simulink model "WIP_2g"  (R2025b)
settings: Solver=ode15s  StartTime=0.0  StopTime=100  MaxStep=1e-2  RelTol=1e-6
InitFcn:
  | run("init.m");
values from neighbouring files (symbols this model uses):
  Fast_Ts = 1e-4    (= 0.0001)    [init.m]
  K1 = robot_params.m1  * robot_params.lc1 + (robot_params.m2 + robot_params.meq)*robot_params.l1    [init.m]
  K2 = robot_params.m2  * robot_params.lc2 + robot_params.meq*robot_params.l2    [init.m]
  q1_init = 0.01; -pi/42;0.01    [init.m]
  q2_init = asin(-K1/K2*sin(q1_init))    [init.m]
undefined symbols (not defined in the file or in its folder): robot_params
settings Model: Creator=Acer  LastModifiedBy=Acer
settings SolverCC: InitialStep=1e-5  SolverResetMethod=Robust

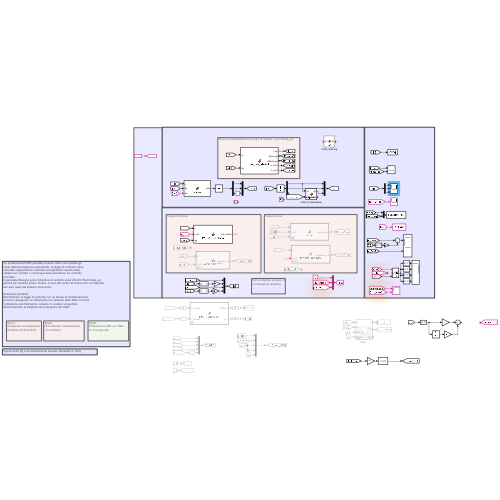
[thumbnail: Simulink's stored preview of the top-level diagram]
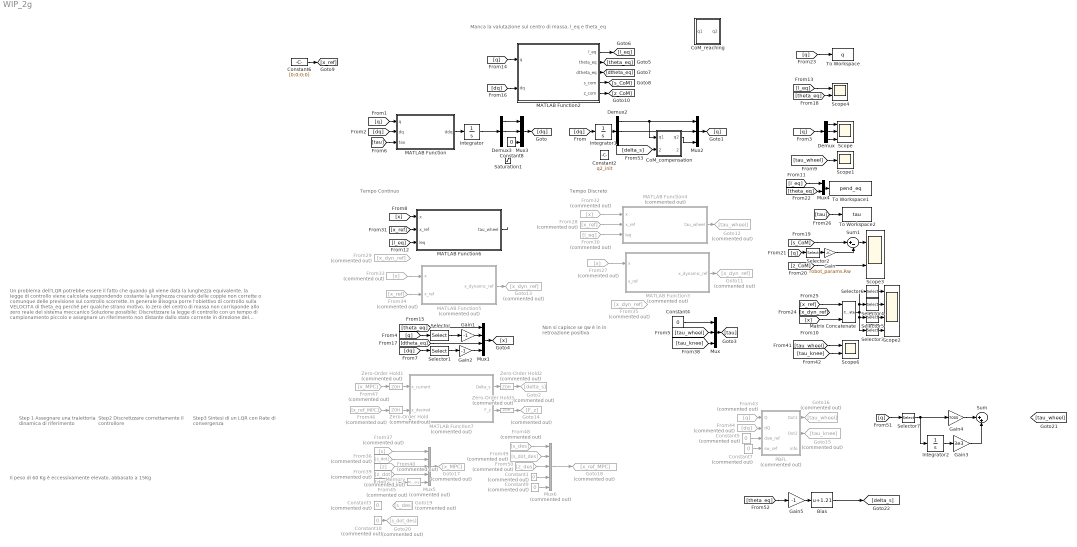
== system WIP_2g ==
  note: Non si capisce se qw è in
      | in retroazione positiva
  note: Il peso di 60 Kg è eccessivamente elevato, abbasato a 15Kg
  note: Tempo Continuo
  note: Step 1
      | Assegnare una traiettoria
      | dinamica di riferimento
  note: Un problema dell'LQR potrebbe essere il fatto che quando gli
      | viene data la lunghezza equivalente, la legge di controllo viene
      | calcolata suppondendo costante la lunghezza creando delle
      | coppie non corrette o comunque delle previsione sul controllo
      | scorrette.
      | In generale Bisogna porre l'obiettivo di controllo sulla VELOCITA di theta_eq
      | perché per qualche strano motivo, lo zero del centro di massa non corrisponde
      | allo zero reale del sistema meccanico
      |
      | Soluzione possibile:
      | Discretizzare la legge di controllo con un tempo di campionamento
      | piccolo e assegnare un riferimento non distante dallo stato corrente
      | in direzione del riferimento costante. In soldoni: progettare
      | dinamicamente la traiettoria da assegnare allo stato
  note: Manca la valutazione sul centro di massa, l_eq e theta_eq
  note: Step2
      | Discretizzare correttamente
      |  il controllore
  note: Tempo Discreto
  note: Step3
      | Sintesi di un LQR con Rate
      | di convergenza
  Bias : Bias  Bias=1.21  SaturateOnIntegerOverflow=off
  CoM_compensation : MATLAB Function  TreatAsAtomicUnit=on
  CoM_reaching : MATLAB Function  TreatAsAtomicUnit=on
  Constant{1,3,5,7,9..10} (6 alike) : Constant  Commented=on  Value=0
  Constant2 : Constant  Value=q2_init
  Constant4 : Constant  Value=0
  Constant6 : Constant  Value=[0;0;0;0]
  Constant8 : Constant  Value=0
  Demux : Demux  Outputs=3
  Demux2 : Demux  Outputs=3
  Demux3 : Demux  Outputs=3
  From27 : From  Commented=on  GotoTag=x
  From28 : From  Commented=on  GotoTag=x_ref
  From29 : From  Commented=on  GotoTag=x_dyn_ref
  From30 : From  Commented=on  GotoTag=l_eq
  From32 : From  Commented=on  GotoTag=x
  From33 : From  Commented=on  GotoTag=x
  From34 : From  Commented=on  GotoTag=x_ref
  From35 : From  Commented=on  GotoTag=x_dyn_ref
  From36 : From  Commented=on  GotoTag=s_dot
  From37 : From  Commented=on  GotoTag=s
  From39 : From  Commented=on  GotoTag=z_dot
  From40 : From  Commented=on  GotoTag=z
  From43 : From  Commented=on  GotoTag=q
  From44 : From  Commented=on  GotoTag=dq
  From45 : From  Commented=on  GotoTag=delta_s
  From46 : From  Commented=on  GotoTag=x_ref_MPC
  From47 : From  Commented=on  GotoTag=x_MPC
  From48 : From  Commented=on  GotoTag=s_des
  From49 : From  Commented=on  GotoTag=s_dot_des
  From50 : From  Commented=on  GotoTag=z_des
  Gain : Gain  Gain=robot_params.Rw
  Gain1 : Gain  Gain=-1
  Gain2 : Gain  Gain=-1
  Gain3 : Gain  Gain=3e3
  Gain4 : Gain  Gain=7000
  Gain5 : Gain  Gain=-1
  Goto11 : Goto  Commented=on  GotoTag=x_dyn_ref
  Goto12 : Goto  Commented=on  GotoTag=tau_wheel
  Goto13 : Goto  Commented=on  GotoTag=x_dyn_ref
  Goto14 : Goto  Commented=on  GotoTag=F_z
  Goto15 : Goto  Commented=on  GotoTag=tau_knee
  Goto16 : Goto  Commented=on  GotoTag=tau_wheel
  Goto17 : Goto  Commented=on  GotoTag=x_MPC
  Goto18 : Goto  Commented=on  GotoTag=x_ref_MPC
  Goto19 : Goto  Commented=on  GotoTag=s_des
  Goto2 : Goto  Commented=on  GotoTag=delta_s
  Goto20 : Goto  Commented=on  GotoTag=s_dot_des
  Integrator : Integrator  InitialCondition=[0;0;0]  ContinuousStateAttributes="\"dq\""
  Integrator1 : Integrator  InitialCondition=[q1_init;0;q2_init]  ContinuousStateAttributes="\"q\""
  Integrator2 : Integrator
  MATLAB Function : MATLAB Function  TreatAsAtomicUnit=on
  MATLAB Function2 : MATLAB Function  TreatAsAtomicUnit=on
  MATLAB Function3 : MATLAB Function  Commented=on  TreatAsAtomicUnit=on  mask{nTs=10, max_amplification=100, min_amplification=1e-3}
  MATLAB Function4 : MATLAB Function  Commented=on  TreatAsAtomicUnit=on
  MATLAB Function5 : MATLAB Function  Commented=on  TreatAsAtomicUnit=on  mask{nTs=1.5, max_amplification=100, min_amplification=1e-3}
  MATLAB Function6 : MATLAB Function  TreatAsAtomicUnit=on  mask{t_settling=10, Q=[1e-10, 1e-10,1e6,1e-3]}
  MATLAB Function7 : MATLAB Function  Commented=on  TreatAsAtomicUnit=on
  Matrix Concatenate : Concatenate  NumInputs=3  Mode=Multidimensional array  ConcatenateDimension=2
  Memory : Memory  Commented=on
  Mux : Mux  Inputs=3
  Mux1 : Mux
  Mux2 : Mux  Inputs=3
  Mux3 : Mux  Inputs=3
  Mux4 : Mux  Inputs=2
  Mux5 : Mux  Commented=on  Inputs=5
  Mux6 : Mux  Commented=on  Inputs=5
  PBFL : Subsystem  Commented=on
  Saturation1 : Saturate  UpperLimit=1  LowerLimit=-1
  Scope : Scope  NumInputPorts=3
      settings: ActiveDisplayString=3  Title=q2  ActiveDisplayYMinimum=1.570486578406654  ActiveDisplayYMaximum=1.5708307432824791
  Scope1 : Scope
      settings: ActiveDisplayYMinimum=-114.88856363268619  ActiveDisplayYMaximum=34.027418421979604
  Scope2 : Scope  NumInputPorts=4
      settings: ActiveDisplayString=4  Title=dqw  ActiveDisplayYMinimum=-52.982971865328068  ActiveDisplayYMaximum=78.205633765029773  DataLoggingVariableName=ScopeData2
  Scope3 : Scope  NumInputPorts=2
      settings: Title=s_CoM - s  ActiveDisplayYMinimum=-0.00016761515520245026  ActiveDisplayYMaximum=1.8924319875646953E-5  DataLoggingVariableName=ScopeData3
  Scope4 : Scope  NumInputPorts=2
      settings: Title=theta_eq  ActiveDisplayYMinimum=-5.3281452597715081E-16  ActiveDisplayYMaximum=4.7823411124945276E-16  DataLoggingVariableName=ScopeData4
  Scope6 : Scope  NumInputPorts=2
      settings: Title=tau_knee  ActiveDisplayYMinimum=-39.904031097666696  ActiveDisplayYMaximum=17.79706307326623  DataLoggingVariableName=ScopeData6
  Selector : Selector  InputPortWidth=3  IndexOptions=Index vector (dialog)  Indices=[2]  OutputSizes=1
  Selector1 : Selector  InputPortWidth=3  IndexOptions=Index vector (dialog)  Indices=[2]  OutputSizes=1
  Selector2 : Selector  InputPortWidth=3  IndexOptions=Index vector (dialog)  Indices=[2]  OutputSizes=1
  Selector3 : Selector  NumberOfDimensions=2  InputPortWidth=3  IndexOptions=Index vector (dialog),Index vector (dialog)  Indices=[4],[1 2 3]  OutputSizes=1,1
  Selector4 : Selector  NumberOfDimensions=2  InputPortWidth=3  IndexOptions=Index vector (dialog),Index vector (dialog)  Indices=[2],[1 2 3]  OutputSizes=1,1
  Selector5 : Selector  NumberOfDimensions=2  InputPortWidth=3  IndexOptions=Index vector (dialog),Index vector (dialog)  Indices=[3],[1 2 3]  OutputSizes=1,1
  Selector6 : Selector  NumberOfDimensions=2  InputPortWidth=3  IndexOptions=Index vector (dialog),Index vector (dialog)  Indices=[1],[1 2 3]  OutputSizes=1,1
  Selector7 : Selector  InputPortWidth=3  IndexOptions=Index vector (dialog)  Indices=1  OutputSizes=1
  Sum : Sum  Inputs=|++
  Sum1 : Sum  Inputs=|+-
  To Workspace : ToWorkspace  VariableName=q  SaveFormat=Timeseries  SampleTime=-1
  To Workspace1 : ToWorkspace  VariableName=pend_eq  SaveFormat=Timeseries  SampleTime=-1
  To Workspace2 : ToWorkspace  VariableName=tau  SaveFormat=Timeseries  SampleTime=-1
  Zero-Order Hold{,1..3} (4 alike) : ZeroOrderHold  Commented=on  SampleTime=1e-2
  wires:
  MATLAB Function/1(ddq) -> Integrator/1
  [dq] -> Integrator1/1
  [q] -> MATLAB Function/1(q)
  [dq] -> MATLAB Function/2(dq)
  Demux/1 -> Scope/1
  [q] -> Demux/1
  Demux/2 -> Scope/2
  [x_ref] -> MATLAB Function6/2(x_ref)
  [l_eq] -> MATLAB Function6/3(leq)
  [tau_wheel] -> Mux/2
  Constant4/1 -> Mux/1
  Mux/1 -> [tau]
  [q] -> Selector/1
  [dq] -> Selector1/1
  Mux1/1 -> [x]
  [x] -> MATLAB Function6/1(x)
  [tau_wheel] -> Scope1/1
  Selector6/1 -> Scope2/1
  Selector4/1 -> Scope2/2
  Selector5/1 -> Scope2/3
  Selector3/1 -> Scope2/4
  [l_eq] -> Scope4/1
  [tau_knee] -> Mux/3
  Demux/3 -> Scope/3
  Integrator1/1 -> Demux2/1
  Mux2/1 -> [q]
  Mux3/1 -> [dq]
  Integrator/1 -> Demux3/1
  [q] -> MATLAB Function2/1(q)
  MATLAB Function2/1(l_eq) -> [l_eq]
  MATLAB Function2/2(theta_eq) -> [theta_eq]
  [theta_eq] -> Mux1/1
  [dq] -> MATLAB Function2/2(dq)
  MATLAB Function2/3(dtheta_eq) -> [dtheta_eq]
  [dtheta_eq] -> Mux1/3
  [theta_eq] -> Scope4/2
  MATLAB Function2/4(s_com) -> [s_CoM]
  MATLAB Function2/5(z_com) -> [z_CoM]
  [s_CoM] -> Sum1/1
  [z_CoM] -> Scope3/2
  [q] -> Selector2/1
  Selector2/1 -> Gain/1
  Gain/1 -> Sum1/2
  Sum1/1 -> Scope3/1
  [theta_eq] -> Mux4/2
  [l_eq] -> Mux4/1
  Mux4/1 -> To Workspace1/1
  [q] -> To Workspace/1
  Constant6/1 -> [x_ref]
  From27/1 -> MATLAB Function3/1(x)
  MATLAB Function3/1(x_dynamic_ref) -> Goto11/1
  [x] -> Matrix Concatenate/3
  [x_ref] -> Matrix Concatenate/1
  Matrix Concatenate/1 -> Selector3/1, Selector5/1, Selector4/1, Selector6/1
  From32/1 -> MATLAB Function4/1(x)
  From30/1 -> MATLAB Function4/3(leq)
  From28/1 -> MATLAB Function4/2(x_ref)
  MATLAB Function5/1(x_dynamic_ref) -> Goto13/1
  From33/1 -> MATLAB Function5/1(x)
  From34/1 -> MATLAB Function5/2(x_ref)
  Selector/1 -> Gain1/1
  Gain1/1 -> Mux1/2
  Selector1/1 -> Gain2/1
  Gain2/1 -> Mux1/4
  ? -> MATLAB Function3/2(x_ref)
  [tau] -> To Workspace2/1
  [tau] -> MATLAB Function/3(tau)
  Demux3/2 -> Mux3/2
  Demux2/2 -> Mux2/2
  MATLAB Function4/1(tau_wheel) -> Goto12/1
  Demux2/1 -> CoM_compensation/1(q1), Mux2/1
  MATLAB Function6/1(tau_wheel) -> ?
  Demux3/1 -> Mux3/1
  [tau_wheel] -> Scope6/1
  [tau_knee] -> Scope6/2
  From43/1 -> PBFL/1(Q)
  From44/1 -> PBFL/2(dQ)
  Constant5/1 -> PBFL/3(dsw_ref)
  Constant7/1 -> PBFL/4(sw_ref)
  PBFL/1(Out1) -> Goto16/1
  PBFL/2(Out2) -> Goto15/1
  Constant8/1 -> Mux3/3
  CoM_compensation/1(q2) -> Mux2/3
  From47/1 -> Zero-Order Hold1/1
  From39/1 -> Mux5/4
  Zero-Order Hold3/1 -> Goto14/1
  Mux6/1 -> Goto18/1
  Memory/1 -> Mux5/5
  From46/1 -> Zero-Order Hold/1
  From48/1 -> Mux6/1
  MATLAB Function7/1(Delta_s) -> Zero-Order Hold2/1
  From50/1 -> Mux6/3
  Constant9/1 -> Mux6/5
  From36/1 -> Mux5/2
  From45/1 -> Memory/1
  From40/1 -> Mux5/3
  Zero-Order Hold1/1 -> MATLAB Function7/1(x_current)
  Zero-Order Hold/1 -> MATLAB Function7/2(x_desired)
  Constant1/1 -> Mux6/4
  From49/1 -> Mux6/2
  MATLAB Function7/2(F_z) -> Zero-Order Hold3/1
  From37/1 -> Mux5/1
  Zero-Order Hold2/1 -> Goto2/1
  Mux5/1 -> Goto17/1
  Constant10/1 -> Goto20/1
  [q] -> Selector7/1
  Gain4/1 -> Sum/1
  Gain3/1 -> Sum/2
  Integrator2/1 -> Gain3/1
  Selector7/1 -> Integrator2/1, Gain4/1
  [theta_eq] -> Gain5/1
  Gain5/1 -> Bias/1
  [delta_s] -> CoM_compensation/2(delta_s)
  Bias/1 -> [delta_s]

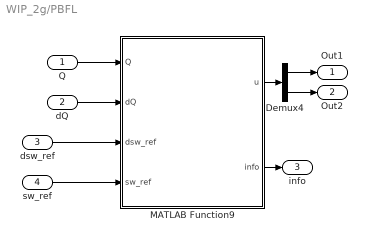
== system WIP_2g/PBFL ==
  Q : Inport
  dQ : Inport  Port=2
  dsw_ref : Inport  Port=3
  sw_ref : Inport  Port=4
  Demux4 : Demux  Outputs=2
  MATLAB Function9 : MATLAB Function  TreatAsAtomicUnit=on
  Out1 : Outport
  Out2 : Outport  Port=2
  info : Outport  Port=3
  wires:
  MATLAB Function9/1(u) -> Demux4/1
  Demux4/1 -> Out1/1
  dQ/1 -> MATLAB Function9/2(dQ)
  Q/1 -> MATLAB Function9/1(Q)
  Demux4/2 -> Out2/1
  MATLAB Function9/2(info) -> info/1
  sw_ref/1 -> MATLAB Function9/4(sw_ref)
  dsw_ref/1 -> MATLAB Function9/3(dsw_ref)

== matlab function WIP_2g/PBFL/MATLAB Function9 ==
  data: Q input; u output; dQ input; dsw_ref input; sw_ref input; info output; gains parameter
function [u, info] = pfl_biped_v3(Q, dQ, dsw_ref, sw_ref, gains)
%#codegen
% Tutti gli stati (Q, dQ) sono quelli reali del plant — nessun ingresso
% "virtuale" separato. theta_ref e' calcolato QUI dentro come funzione di
% qw, dqw, non e' un riferimento esterno fornito dall'utente.
%
% gains = [kp1; kd1; kp_pc; kd_pc; kv; kx; theta_max; pc_max; tau_max]

    Rw = 0.127;
    m1=1.2; m2=5.3; meq=15.0; l1=0.45; l2=0.45; lc1=l1/2; lc2=l2/2;
    K1 = m1*lc1 + (m2+meq)*l1;
    K2 = m2*lc2 + meq*l2;
    mtot = 3.5 + m1 + m2 + meq;

    kp1=gains(1); kd1=gains(2);
    kp_pc=gains(3); kd_pc=gains(4);
    kv=gains(5); kx=gains(6);
    theta_max=gains(7); pc_max=gains(8); tau_max=gains(9);

    q1=Q(1); qw=Q(2); q2=Q(3);
    dq1=dQ(1); dqw=dQ(2); dq2=dQ(3);
    c1=cos(q1); s1=sin(q1); c2=cos(q2); s2=sin(q2);

    [M,~,CdQ,G,B] = calc_dynamics(Q,dQ);
    h = CdQ + B*dQ + G;
    S = [-1,-1; 1,0; 0,1];

    % --- riferimento di postura DERIVATO dagli stati reali qw, dqw -------
    sw  = Rw*qw;
    dsw = Rw*dqw;
    theta_ref = -kv*(dsw - dsw_ref) - kx*(sw - sw_ref);
    theta_ref = sat(theta_ref, theta_max);

    % --- uscita 1: postura, ora rincorre theta_ref invece di una costante
    v1 = -kp1*(q1 - theta_ref) - kd1*dq1;

    % --- uscita 2: bilanciamento CoM, invariata -----------------------
    pc  = (K1*s1 + K2*s2)/mtot;
    dpc = (K1*c1*dq1 + K2*c2*dq2)/mtot;
    drift = -(K1*s1*dq1^2 + K2*s2*dq2^2)/mtot;
    pc_ref = sat(0, pc_max);   % qui puoi tenerlo a 0, il bilanciamento resta locale
    v2 = -kp_pc*(pc - pc_ref) - kd_pc*dpc;

    A = [1,0,0; K1*c1/mtot,0,K2*c2/mtot];
    D = A*(M\S);
    rhs = [v1; v2 - drift] + A*(M\h);

    u = D \ rhs;
    u = [sat(u(1),tau_max); sat(u(2),tau_max)];

    info = [theta_ref; pc; sw; dsw];
end

function y = sat(x,lim)
    y = min(max(x,-lim),lim);
end

== matlab function WIP_2g/MATLAB Function7 ==
  data: x_current input; Delta_s output; x_desired input; F_z output
function [Delta_s, F_z] = MPC_Custom_QP(x_current, x_desired)
    % quadprog non è supportato nativamente per la code generation C
    coder.extrinsic('quadprog');
    coder.extrinsic('optimoptions');

    %% 1. Parametri e Discretizzazione
    m_b = 73.0; 
    g = 9.81;    
    
    h = x_current(3); 
    if h < 0.1
        h = 0.6;
    end
    
    dt = 0.01; 
    N = 40;     
    
    A_c = zeros(5,5);
    A_c(1,2) = 1;
    A_c(3,4) = 1;
    A_c(2,5) = g / h; 
    
    B_c = zeros(5,2);
    B_c(4,2) = 1 / m_b;
    B_c(5,1) = 1;
    
    A_d = eye(5) + A_c * dt;
    B_d = B_c * dt;

    %% 2. Pesi della Funzione di Costo
    %x = [s, ṡ, z, ż, Δs]
    S = diag([1, 1, 500, 50, 1]);
    W = diag([1, 0.01]);

    %% 3. Condensazione (Srotolamento) 
    nx = 5; nu = 2;
    P_x = zeros(nx*N, nx);
    P_u = zeros(nx*N, nu*N);

    A_power = eye(nx);
    for i = 1:N
        A_power = A_power * A_d;
        P_x((i-1)*nx+1 : i*nx, :) = A_power;
        for j = 1:i
            P_u((i-1)*nx+1 : i*nx, (j-1)*nu+1 : j*nu) = (A_d^(i-j)) * B_d;
        end
    end

    S_bar = kron(eye(N), S);
    W_bar = kron(eye(N), W);

    H = 2 * (P_u' * S_bar * P_u + W_bar);
    H = (H + H') / 2; % Garantisce simmetria perfetta
    
    X_ref = repmat(x_desired, N, 1);
    f = 2 * P_u' * S_bar * (P_x * x_current - X_ref);

    %% 4. Vincoli Fisici
    F_min = -1500; % Permette di frenare!
    F_max = 1500;
    
    LB = zeros(nu*N, 1);
    UB = zeros(nu*N, 1);
    
    for i = 1:N
        LB((i-1)*nu+1) = -0.20;   % era -2.0

        UB((i-1)*nu+1) =  0.20;   % era  2.0
 
        
        LB((i-1)*nu+2) = F_min; 
        UB((i-1)*nu+2) = F_max;
    end

    %% 5. Risoluzione QP (CORRETTA)
    % Pre-allocazione per Simulink Coder
    U_opt_calc = zeros(nu*N, 1);
    fval = 0.0;
    exitflag = 0.0;
    
    % Algoritmo robusto di default
    options = optimoptions('quadprog', 'Display', 'off');
    
    % LA CORREZIONE: Aggiunto "fval" per non sballare "exitflag"!
    [U_opt_calc, fval, exitflag] = quadprog(H, f, [], [], [], [], LB, UB, [], options);

    if exitflag > 0
        U_opt = U_opt_calc;
    else
        % Se fallisce davvero, eroga 0 extra, ma il VMC ci terrà in piedi col peso base
        U_opt = zeros(nu*N, 1);
    end

    %% 6. Estrazione Input Ottimo
    Delta_s_dot_opt = U_opt(1);
    F_z = U_opt(2); % FINALMENTE SARA' DIVERSO DA ZERO!

    Delta_s = x_current(5) + Delta_s_dot_opt * dt;
end

== matlab function WIP_2g/MATLAB Function ==
  settings: updateMethod=CONTINUOUS
  data: q input double size=3; dq input double size=3; tau input size=3; ddq output double size=3; robot_params parameter
function ddq = Dynamics(q,dq,tau,robot_params)


q1 = q(1);
qw = q(2);
q2 = q(3);
dq1 = dq(1);
dqw = dq(2);
dq2 = dq(3);

m1 = robot_params.m1;
m2 = robot_params.m2;
meq = robot_params.meq;
lc2 = robot_params.lc1;
lc1 = robot_params.lc2;
l1 = robot_params.l1;
l2 = robot_params.l2;
mw = robot_params.mw;
Rw = robot_params.Rw;
Iw= robot_params.Iw;
g = robot_params.g;
bw =  robot_params.bw;
b1 =  robot_params.b1;
b2 = robot_params.b2;
I1 = robot_params.I1;  
I2 = robot_params.I2;



M = [ I1 + l1^2*m2 + lc1^2*m1 + l1^2*meq,        Rw*cos(q1)*(l1*m2 + lc1*m1 + l1*meq), l1*cos(q1 - q2)*(lc2*m2 + l2*meq);
      Rw*cos(q1)*(l1*m2 + lc1*m1 + l1*meq), Iw + Rw^2*m1 + Rw^2*m2 + Rw^2*meq + Rw^2*mw,      Rw*cos(q2)*(lc2*m2 + l2*meq);
       l1*cos(q1 - q2)*(lc2*m2 + l2*meq),                Rw*cos(q2)*(lc2*m2 + l2*meq),          meq*l2^2 + m2*lc2^2 + I2];

 C = [ 0, 0, dq2*l1*sin(q1 - q2)*(lc2*m2 + l2*meq);
    -Rw*dq1*sin(q1)*(l1*m2 + lc1*m1 + l1*meq), 0,     -Rw*dq2*sin(q2)*(lc2*m2 + l2*meq);
     -dq1*l1*sin(q1 - q2)*(lc2*m2 + l2*meq), 0, 0];
 
B = [b1,  0,  0;
   0, bw,  0;
   0,  0, b2];

G = [-g*sin(q1)*(l1*m2 + lc1*m1 + l1*meq);
                                   0;
        -g*sin(q2)*(lc2*m2 + l2*meq)];
 

ddq = M\(-(C+B)*dq -G + tau);

== matlab function WIP_2g/MATLAB Function2 ==
  data: q input; dq input; l_eq output; theta_eq output; dtheta_eq output; robot_params parameter; s_com output; z_com output
function [l_eq, theta_eq, dtheta_eq, s_com, z_com] = calc_com_simulink(q, dq, robot_params)
% CALC_COM_SIMULINK  MATLAB Function block per Simulink.
% Calcola CoM globale, pendolo equivalente e derivate temporali.
%
% Input:
%   q            : [3x1] — [q1; qw; q2]  coordinate generalizzate [rad]
%   dq           : [3x1] — [dq1; dqw; dq2] velocita' generalizzate [rad/s]
%   robot_params : struct con campi .mw .Rw .m1 .m2 .meq .l1 .l2 .lc1 .lc2
%
% Output:
%   x_com     : coordinata x CoM globale [m]
%   y_com     : coordinata y CoM globale [m]
%   l_eq      : distanza centro ruota — CoM [m]
%   theta_eq  : angolo pendolo equivalente dalla verticale [rad], zero quando CoM e' sopra il pivot
%   dl_eq     : d/dt(l_eq)     [m/s]
%   dtheta_eq : d/dt(theta_eq) [rad/s]

% -------------------------------------------------------------------------
% Parametri
% -------------------------------------------------------------------------
Rw  = robot_params.Rw;
m1  = robot_params.m1;
m2  = robot_params.m2;
meq = robot_params.meq;
l1  = robot_params.l1;
l2  = robot_params.l2;
lc1 = robot_params.lc1;
lc2 = robot_params.lc2;
M_tot = m1 + m2 + meq;

% -------------------------------------------------------------------------
% Coordinate e velocita'
% -------------------------------------------------------------------------
q1 = q(1);  dq1 = dq(1);
qw = q(2);  dqw = dq(2);
q2 = q(3);  dq2 = dq(3);

sw  = Rw * qw;
dsw = Rw * dqw;   % d/dt(sw)

% -------------------------------------------------------------------------
% Posizioni CoM parziali
% -------------------------------------------------------------------------
x_c1 = sw  + lc1*sin(q1);
y_c1 = Rw  + lc1*cos(q1);

xk   = sw  + l1*sin(q1);
yk   = Rw  + l1*cos(q1);

x_c2 = xk  + lc2*sin(q2);
y_c2 = yk  + lc2*cos(q2);

xh   = xk  + l2*sin(q2);
yh   = yk  + l2*cos(q2);

% -------------------------------------------------------------------------
% Velocita' CoM parziali — derivata temporale diretta
% -------------------------------------------------------------------------
dx_c1 = dsw + lc1*cos(q1)*dq1;
dy_c1 =     - lc1*sin(q1)*dq1;

dxk   = dsw + l1*cos(q1)*dq1;
dyk   =     - l1*sin(q1)*dq1;

dx_c2 = dxk + lc2*cos(q2)*dq2;
dy_c2 = dyk - lc2*sin(q2)*dq2;

dxh   = dxk + l2*cos(q2)*dq2;
dyh   = dyk - l2*sin(q2)*dq2;

% -------------------------------------------------------------------------
% CoM globale e sua velocita'
% -------------------------------------------------------------------------
x_com  = (m1*x_c1  + m2*x_c2  + meq*xh)  / M_tot;
y_com  = (m1*y_c1  + m2*y_c2  + meq*yh)  / M_tot;

s_com = x_com;
z_com = y_com;

dx_com = (m1*dx_c1 + m2*dx_c2 + meq*dxh) / M_tot;
dy_com = (m1*dy_c1 + m2*dy_c2 + meq*dyh) / M_tot;

% -------------------------------------------------------------------------
% Pendolo equivalente — pivot in (sw, Rw)
% -------------------------------------------------------------------------
dx = x_com - sw;
dy = y_com - Rw;

% Derivate temporali di dx e dy
ddx = dx_com - dsw;
ddy = dy_com;        % Rw costante

l_eq     = sqrt(dx^2 + dy^2);
theta_eq = atan2(dx, dy);

% d/dt(l_eq)     = (dx*ddx + dy*ddy) / l_eq
% d/dt(theta_eq) = (dy*ddx - dx*ddy) / l_eq^2
dl_eq     = (dx*ddx + dy*ddy) / l_eq;
dtheta_eq = (dy*ddx - dx*ddy) / (l_eq^2);

end

== matlab function WIP_2g/MATLAB Function3 ==
  settings: updateMethod=DISCRETE  sampleTime=Fast_Ts
  data: x input double size=4; x_dynamic_ref output double size=4; x_ref input double size=4; nTs parameter; min_amplification parameter; max_amplification parameter
function x_dynamic_ref  = Dynamic_trajectory(x, x_ref, nTs,min_amplification, max_amplification)

%% Input
% x stato attuale
% x_ref stato di riferimento a regime

%% Output
% x_dynamic_ref inteso come traiettoria da dare dinamicamente come
% riferimento al controllo LQR

x_dynamic_ref = zeros(4,1);

%% Parameter
% nTs numero di passi entro cui raggiungere il regime
% Fast_Ts frequenza di campionamento

%% Codice
min_amplification; % quando err_theta_eq = 0;
max_amplification ; % quando err_theta_eq = 2pi;

a = min_amplification;
b = max_amplification;
err_theta_eq = abs(x_ref(3) - x(3))*abs(x(3));

G_lin = (a-sign(err_theta_eq)*err_theta_eq/2/pi * (a - b))*sign(err_theta_eq);

G_quad =a/[(1 + sign(err_theta_eq)*err_theta_eq/2/pi*(1/b-1))*((1 + sign(err_theta_eq)*err_theta_eq/2/pi*(a-1)))]*sign(err_theta_eq);

Delta_x = x_ref - x;

n_amplified  = nTs/G_lin;



x_dynamic_ref(3) = x(3) + 1/n_amplified*(Delta_x(3));
%x_dynamic_ref(3) = x(3) + 1/nTs*(Delta_x(3));
x_dynamic_ref(1:2) = x(1:2) + 1/nTs.*(Delta_x(1:2));
x_dynamic_ref(4) = x(4) + 1/nTs.*(Delta_x(4));

== matlab function WIP_2g/MATLAB Function4 ==
  settings: updateMethod=DISCRETE  sampleTime=Fast_Ts
  data: x input double size=4; tau_wheel output; x_ref input double size=4; leq input double size=1; robot_params parameter; Fast_Ts parameter
function tau_wheel = TV_DLQR_2D(x, x_ref, leq, robot_params, Fast_Ts)
    % x: Stato attuale [s; theta; s_dot; theta_dot;] (4x1)
    % x_ref: Stato target desiderato (deve avere almeno 4 elementi per combaciare con x)
    % leq: Lunghezza attuale del pendolo equivalente [m]
    % robot_params: Struttura dei parametri fisici
    % Ts: Tempo di campionamento [s]
    
    % Dichiara funzioni esterne per la generazione codice in Simulink
    coder.extrinsic('dlqr', 'expm');
    

    Ts = Fast_Ts;
    % Estrazione parametri fisici
    m_eq = robot_params.meq + robot_params.m1 + robot_params.m2;
    mw = robot_params.mw;
    Rw = robot_params.Rw;
    Iw = robot_params.Iw;
    g = robot_params.g;
    bw = robot_params.bw;
    
    % Evita divisioni per zero al primo step di simulazione o per leq nullo
    if leq < 1e-4
        leq = 1e-4;
    end
    
    % Matrici a tempo continuo (Sistema \dot{x} = Ax + Bu)
    A = [0, 0, 1, 0;
         0, 0, 0, 1;
        (g*(Iw + Rw^2*m_eq + Rw^2*mw))/(leq*(mw*Rw^2 + Iw)), 0, 0, (Rw*bw)/(leq*(mw*Rw^2 + Iw));
        -(Rw*g*m_eq)/(mw*Rw^2 + Iw), 0, 0, -bw/(mw*Rw^2 + Iw)];
 
    B = [0; 0; -Rw/(leq*(mw*Rw^2 + Iw)); 1/(mw*Rw^2 + Iw)];
    
    % ---------------------------------------------------------
    % DISCRETIZZAZIONE ZOH (Zero-Order Hold)
    % ---------------------------------------------------------
    % Costruisce la matrice aumentata [A, B; 0, 0] per l'esponenziale
    M_cont = [A, B; zeros(1, 5)];
    
    % Inizializza matrici per Code Gen
    Ad = zeros(4, 4);
    Bd = zeros(4, 1);
    
    % Calcola esatto ZOH tramite expm 
    M_disc = expm(M_cont * Ts);
    
    Ad = M_disc(1:4, 1:4);
    Bd = M_disc(1:4, 5);
    
    % NOTA: Per tempi di campionamento estremamente bassi (es. Ts = 0.001) 
    % e per risparmiare costo computazionale real-time, potresti usare 
    % l'approssimazione di Eulero in avanti:
    % Ad = eye(4) + A * Ts;
    % Bd = B * Ts;
    
    % ---------------------------------------------------------
    % PROGETTO LQR DISCRETO
    % ---------------------------------------------------------
    % Matrici di peso
    % [theta_eq, qw, dot_theta_eq, dot_qw]
    Q = diag([1e1, 1e-6, 1e5, 1]);
    R = 1e-2; 
    
    % Inizializza K per la Code Generation di Simulink
    K = zeros(1, 4); 
    
    % Calcola la matrice dei guadagni ottimali K tramite dlqr
    K = dlqr(Ad, Bd, Q, R);
    
    % Assicura dimensioni compatibili: x è 4x1, x_ref potrebbe essere 6x1 dal tuo commento.
    % Tronchiamo x_ref ai primi 4 elementi di interesse se necessario.
    if length(x_ref) > 4
        x_ref_LQR = x_ref(1:4);
    else
        x_ref_LQR = x_ref;
    end
    
    % Errore di stato (tilde_X)
    x_tilde = x - x_ref_LQR;
    
    % Legge di controllo per il tempo discreto
    tau_wheel = -K * x_tilde; 
end

== matlab function WIP_2g/MATLAB Function5 ==
  settings: updateMethod=CONTINUOUS  sampleTime=Fast_Ts
  data: x input double size=4; x_dynamic_ref output double size=4; x_ref input double size=4; nTs parameter; min_amplification parameter; max_amplification parameter
function x_dynamic_ref  = Dynamic_trajectory(x, x_ref, nTs,min_amplification, max_amplification)

%% Input
% x stato attuale
% x_ref stato di riferimento a regime

%% Output
% x_dynamic_ref inteso come traiettoria da dare dinamicamente come
% riferimento al controllo LQR

x_dynamic_ref = zeros(4,1);

%% Parameter
% nTs numero di passi entro cui raggiungere il regime
% Fast_Ts frequenza di campionamento

%% Codice
min_amplification; % quando err_theta_eq = 0;
max_amplification ; % quando err_theta_eq = 2pi;

a = min_amplification;
b = max_amplification;
err_theta_eq = abs(x_ref(3) - x(3))*abs(x(3));

G_lin = (a-sign(err_theta_eq)*err_theta_eq/2/pi * (a - b))*sign(err_theta_eq);

G_quad =a/[(1 + sign(err_theta_eq)*err_theta_eq/2/pi*(1/b-1))*((1 + sign(err_theta_eq)*err_theta_eq/2/pi*(a-1)))]*sign(err_theta_eq);

Delta_x = x_ref - x;

n_amplified  = nTs/G_lin;



%x_dynamic_ref(3) = x(3) + 1/n_amplified*(Delta_x(3));
if( abs(x(3) + 1/nTs*(Delta_x(3)))<1e-4)
    x_dynamic_ref(3) = 0;
else
    x_dynamic_ref(3) = x(3) + 1/nTs*(Delta_x(3));
end
x_dynamic_ref(1:2) = x(1:2) + 1/nTs.*(Delta_x(1:2));
x_dynamic_ref(4) = x(4) + 1/nTs.*(Delta_x(4));

== matlab function WIP_2g/MATLAB Function6 ==
  data: x input double size=4; tau_wheel output; x_ref input double size=4; leq input double size=1; robot_params parameter; t_settling parameter; Q parameter
function tau_wheel  = TV_LQR_2D_alpha(x, x_ref, leq, robot_params, t_settling,Q)
    % x: Stato attuale [s; theta;  s_dot; theta_dot; ] (4x1)
    % x_ref: Stato target desiderato (4x1)
    % leq: Lunghezza attuale del pendolo equivalente [m]
    % robot_params: Struttura con i parametri del robot
    % t_settling: Tempo di assestamento desiderato [s] (criterio del 2%)
    
    coder.extrinsic('lqr');
    
    % Estrazione parametri
    m_eq = robot_params.meq + robot_params.m1 + robot_params.m2;
    mw = robot_params.mw;
    Rw = robot_params.Rw;
    Iw= robot_params.Iw;
    g = robot_params.g;
    bw =  robot_params.bw;
    
    % Evita divisioni per zero al primo step di simulazione
    if leq < 1e-4
        leq = 1e-4;
    end
    
    % Matrici del sistema lineare
    A = [0, 0, 1, 0;
         0, 0, 0, 1;
        (g*(Iw + Rw^2*m_eq + Rw^2*mw))/(leq*(mw*Rw^2 + Iw)), 0, 0, (Rw*bw)/(leq*(mw*Rw^2 + Iw));
        -(Rw*g*m_eq)/(mw*Rw^2 + Iw), 0, 0, -bw/(mw*Rw^2 + Iw)];
 
    B = [0; 0; -Rw/(leq*(mw*Rw^2 + Iw)); 1/(mw*Rw^2 + Iw)];
    
    % Pesi per l'LQR
    Q_theta_eq = Q(1);
    Q_qw= Q(2);
    Q_dot_theta_eq= Q(3);
    Q_dot_qw = Q(4);
    %[1e3, 1e-4,1e3,1e3]
    Q = diag([Q_theta_eq, Q_qw, Q_dot_theta_eq, Q_dot_qw]);
    R = 0.001;         
    
    % ---------------------------------------------------------
    % IMPLEMENTAZIONE ALPHA-SHIFT (Grado di stabilità prescritto)
    % ---------------------------------------------------------
    % Calcola il rate di convergenza alpha in base al tempo di assestamento
    % Protezione per evitare divisioni per zero se t_settling è 0
    if t_settling < 0.01
        t_settling = 0.01; 
    end
    alpha = 4.0 / t_settling;
    
    % Trasla la matrice A
    A_alpha = A + alpha * eye(4);
    
    % Risoluzione LQR con la matrice traslata
    K = zeros(1, 4); 
    K = lqr(A_alpha, B, Q, R);
    
    % Errore di stato
    x_tilde = x - x_ref;
    
    % Calcolo della coppia
    tau_wheel = -K * x_tilde; 
end

== matlab function WIP_2g/CoM_reaching ==
  data: q1 input; q2 output; K1 parameter; K2 parameter
function q2= fcn(q1,K1, K2)

q2 = real(asin(-K1/K2*sin(q1)));

== matlab function WIP_2g/CoM_compensation ==
  data: q1 input; q2 output; robot_params parameter; is_feasible output; delta_s input
function [q2, is_feasible] = compute_q2_with_offset(q1, robot_params, delta_s)
% COMPUTE_Q2_WITH_OFFSET Calcola l'angolo q2 necessario per ottenere un
% offset orizzontale delta_s del CoM rispetto al centro della ruota.
% 
% Input:
%   q1           : Angolo del primo giunto [rad]
%   delta_s      : Offset desiderato (x_com - sw) [m]. 
%                  (delta_s = 0 equivale a theta_eq = 0)
%   robot_params : Struct con i parametri di massa e lunghezza del robot
%
% Output:
%   q2           : Angolo calcolato per il secondo giunto [rad]
%   is_feasible  : Booleano, true se la postura è fisicamente raggiungibile

    % 1. Estrazione parametri
    m1  = robot_params.m1;
    m2  = robot_params.m2;
    meq = robot_params.meq;
    l1  = robot_params.l1;
    lc1 = robot_params.lc1;
    l2  = robot_params.l2; 
    lc2 = robot_params.lc2;
    
    % 2. Massa totale
    M_tot = m1 + m2 + meq;
    
    % 3. Calcolo costanti di aggregazione dei bracci (Momenti statici relativi)
    % K1: Contributo del primo link e delle masse a valle
    K1 = m1*lc1 + m2*l1 + meq*l1;
    
    % K2: Contributo del secondo link e della massa equivalente in cima
    K2 = m2*lc2 + meq*l2;
    
    % 4. Calcolo del valore richiesto per il seno di q2
    sin_q2_req = (M_tot * delta_s - K1 * sin(q1)) / K2;
    
    % 5. Verifica di fattibilità cinematica e calcolo di q2
    if abs(sin_q2_req) > 1
        is_feasible = false;
        % Satura al limite fisico (braccio esteso al massimo in orizzontale)
        q2 = sign(sin_q2_req) * (pi / 2); 
    else
        is_feasible = true;
        q2 = asin(sin_q2_req);
    end
end
